simulink model "method3"  (R2025a)
settings: Solver=ode45  StartTime=0.0  StopTime=100  MaxStep=0.001  RelTol=1e-3
settings Model: Creator=vm66c  LastModifiedBy=vm66c

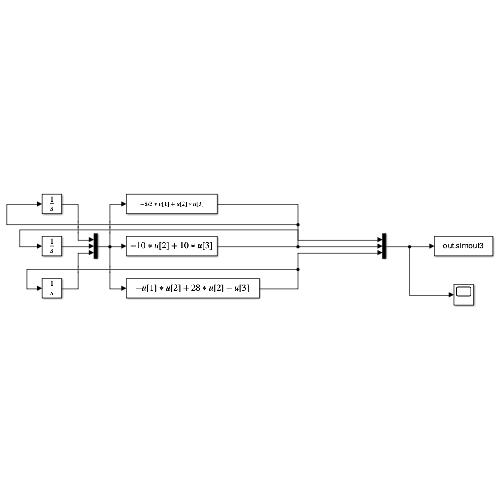
[thumbnail: Simulink's stored preview of the top-level diagram]
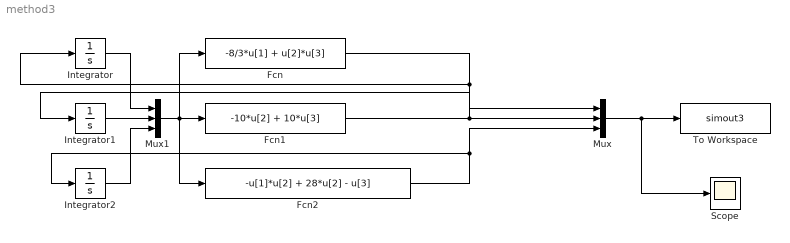
== system method3 ==
  Fcn : Fcn  Expr=-8/3*u[1] + u[2]*u[3]
  Fcn1 : Fcn  Expr=-10*u[2] + 10*u[3]
  Fcn2 : Fcn  Expr=-u[1]*u[2] + 28*u[2] - u[3]
  Integrator : Integrator
  Integrator1 : Integrator
  Integrator2 : Integrator  InitialCondition=1e-10
  Mux : Mux  Inputs=3
  Mux1 : Mux  Inputs=3
  Scope : Scope
      settings: ActiveDisplayYMinimum=-488.1887862457873  ActiveDisplayYMaximum=509.15939201454177
  To Workspace : ToWorkspace  VariableName=simout3  SampleTime=-1
  wires:
  Integrator1/1 -> Mux1/2
  Integrator/1 -> Mux1/1
  Integrator2/1 -> Mux1/3
  Mux1/1 -> Fcn2/1, Fcn/1, Fcn1/1
  Fcn/1 -> Mux/1, Integrator/1
  Fcn1/1 -> Mux/2, Integrator1/1
  Fcn2/1 -> Mux/3, Integrator2/1
  Mux/1 -> Scope/1, To Workspace/1
